simulink model "Prvi"  (R2020a)
settings: Solver=VariableStepAuto  StartTime=0.0  StopTime=100  RelTol=1e-3
settings Model: Creator=Aldin  LastModifiedBy=Aldin

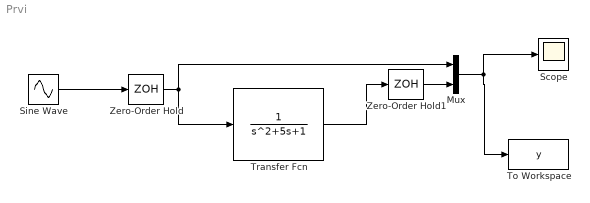
== system Prvi ==
  Mux : Mux  Inputs=2
  Scope : Scope
  Sine Wave : Sin  Amplitude=4  Frequency=0.25  SampleTime=0.1
  To Workspace : ToWorkspace  VariableName=y  SampleTime=-1
  Transfer Fcn : TransferFcn  Denominator=[1 5 1]
  Zero-Order Hold : ZeroOrderHold  SampleTime=0.1
  Zero-Order Hold1 : ZeroOrderHold  SampleTime=0.1
  wires:
  Zero-Order Hold/1 -> Mux/1, Transfer Fcn/1
  Mux/1 -> To Workspace/1, Scope/1
  Zero-Order Hold1/1 -> Mux/2
  Transfer Fcn/1 -> Zero-Order Hold1/1
  Sine Wave/1 -> Zero-Order Hold/1
